simulink model "RobotX_September11"  (R2014a)
settings: Solver=FixedStepDiscrete  StartTime=0.0  StopTime=inf  FixedStep=.1  RelTol=1e-3
undefined symbols (not defined in the file): Com1, Com2, Com3, Com4, DiscIntNeverNeededParam
libraries: xpcseriallib x8, simulink x2, speedgoatlib_IO102 x1, slrtlib x1
(part 1 of 2)
settings Model: BufferReuse=off  Creator=wildcat  LastModifiedBy=wildcat
settings SolverCC: EnableConcurrentExecution=on
settings DataIOCC: SignalLoggingSaveFormat=ModelDataLogs
settings OptimizationCC: BlockReduction=off  OptimizeBlockIOStorage=off  BufferReuse=off  GlobalBufferReuse=off  ExpressionFolding=off  LocalBlockOutputs=off
settings DebuggingCC: UnderspecifiedInitializationDetection=Classic  StateNameClashWarn=warning
settings HardwareCC: ProdIntDivRoundTo=Zero  ProdEndianess=LittleEndian  ProdHWDeviceType=Generic->32-bit x86 compatible
settings RTWCC: SystemTargetFile=slrt.tlc  TemplateMakefile=slrt_default_tmf  Description=Simulink Real-Time  ProcessScript=slrt_make_rtw_hook  RTWCompilerOptimization=On
settings SimulinkRealTimeCC: GeneratePreprocessorConditionals=Disable all  EnableShiftOperators=on

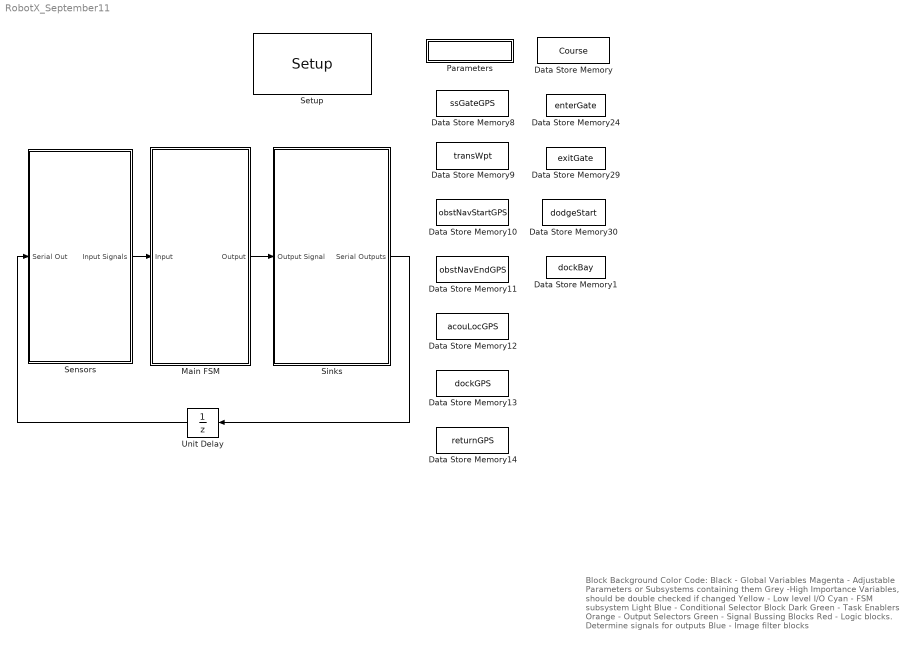
== system RobotX_September11 ==
  note: Block Background Color Code:
      | Black - Global Variables
      | Magenta - Adjustable Parameters or Subsystems containing them
      | Grey -High Importance Variables, should be double checked if changed
      | Yellow - Low level I/O
      | Cyan - FSM subsystem
      | Light Blue - Conditional Selector Block
      | Dark Green - Task Enablers
      | Orange - Output Selectors
      | Green - Signal Bussing Blocks
      | Red - Logic blocks. Determine signals for outputs
      | Blue - Image filter blocks
  Data Store Memory : DataStoreMemory  DataStoreName=Course  ReadBeforeWriteMsg=warning  WriteAfterWriteMsg=warning  WriteAfterReadMsg=warning
  Data Store Memory1 : DataStoreMemory  DataStoreName=dockBay  ReadBeforeWriteMsg=warning  WriteAfterWriteMsg=warning  WriteAfterReadMsg=warning
  Data Store Memory10 : DataStoreMemory  DataStoreName=obstNavStartGPS  ReadBeforeWriteMsg=warning  WriteAfterWriteMsg=warning  WriteAfterReadMsg=warning  InitialValue=zeros(1,2)
  Data Store Memory11 : DataStoreMemory  DataStoreName=obstNavEndGPS  ReadBeforeWriteMsg=warning  WriteAfterWriteMsg=warning  WriteAfterReadMsg=warning  InitialValue=zeros(1,2)
  Data Store Memory12 : DataStoreMemory  DataStoreName=acouLocGPS  ReadBeforeWriteMsg=warning  WriteAfterWriteMsg=warning  WriteAfterReadMsg=warning  InitialValue=zeros(1,2)
  Data Store Memory13 : DataStoreMemory  DataStoreName=dockGPS  ReadBeforeWriteMsg=warning  WriteAfterWriteMsg=warning  WriteAfterReadMsg=warning  InitialValue=zeros(1,2)
  Data Store Memory14 : DataStoreMemory  DataStoreName=returnGPS  ReadBeforeWriteMsg=warning  WriteAfterWriteMsg=warning  WriteAfterReadMsg=warning  InitialValue=zeros(1,2)
  Data Store Memory24 : DataStoreMemory  DataStoreName=enterGate  ReadBeforeWriteMsg=warning  WriteAfterWriteMsg=warning  WriteAfterReadMsg=warning
  Data Store Memory29 : DataStoreMemory  DataStoreName=exitGate  ReadBeforeWriteMsg=warning  WriteAfterWriteMsg=warning  WriteAfterReadMsg=warning
  Data Store Memory30 : DataStoreMemory  DataStoreName=dodgeStart  ReadBeforeWriteMsg=warning  WriteAfterWriteMsg=warning  WriteAfterReadMsg=warning
  Data Store Memory8 : DataStoreMemory  DataStoreName=ssGateGPS  ReadBeforeWriteMsg=warning  WriteAfterWriteMsg=warning  WriteAfterReadMsg=warning  InitialValue=zeros(1,2)
  Data Store Memory9 : DataStoreMemory  DataStoreName=transWpt  ReadBeforeWriteMsg=warning  WriteAfterWriteMsg=warning  WriteAfterReadMsg=warning  InitialValue=zeros(1,2)
  Main FSM : Subsystem
  Parameters : Subsystem
  Sensors : Subsystem
  Setup : speedgoatlib_IO102/Setup  group=Digital output setup  id=1  range=+-5V  cal=off  pciSlot=-1  adChannelMode=Multiple-channel (enter number of channels below)  adChannel=16  adCoupling=Differential  daChannel=[1,2,3,4]  daReset=[1]  daInitValue=[0]  diChannel=[1,2,3,4,5,6,7,8]  doChannel=[1,2,3,4,5,6,7,8]  doReset=[1]  doInitValue=[0]
  Sinks : Subsystem
  Unit Delay : UnitDelay  SampleTime=-1
  wires:
  Main FSM/1(Output) -> Sinks/1(Output Signal)
  Sensors/1(Input Signals) -> Main FSM/1(Input)
  Sinks/1(Serial Outputs) -> Unit Delay/1
  Unit Delay/1 -> Sensors/1(Serial Out)

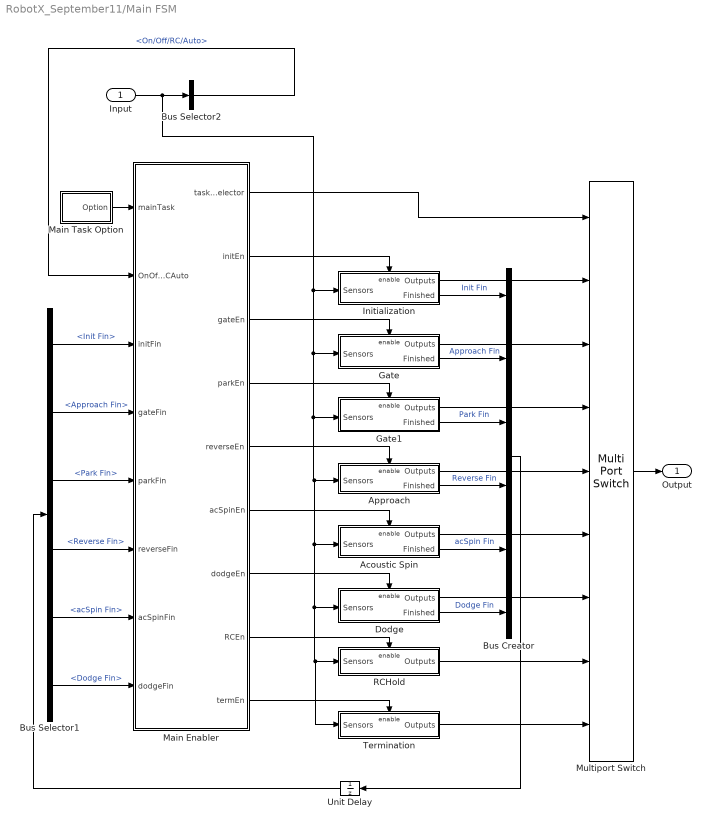
== system RobotX_September11/Main FSM ==
  Input : Inport
  Acoustic Spin : Subsystem  TreatAsAtomicUnit=on
  Approach : Subsystem  TreatAsAtomicUnit=on
  Bus Creator : BusCreator  Inputs=6
  Bus Selector1 : BusSelector  OutputSignals=Init Fin,Approach Fin,Park Fin,Reverse Fin,acSpin Fin,Dodge Fin
  Bus Selector2 : BusSelector  OutputSignals=LCM Message.On/Off/RC/Auto
  Dodge : Subsystem  TreatAsAtomicUnit=on
  Gate : Subsystem  TreatAsAtomicUnit=on
  Gate1 : Subsystem  TreatAsAtomicUnit=on
  Initialization : Subsystem
  Main Enabler : MATLAB Function  TreatAsAtomicUnit=on
  Main Task Option : Subsystem
  Multiport Switch : MultiPortSwitch  Inputs=8
  RCHold : Subsystem
  Termination : Subsystem  TreatAsAtomicUnit=on
  Unit Delay : UnitDelay  SampleTime=-1
  Output : Outport
  wires:
  Main Task Option/1(Option) -> Main Enabler/1(mainTask)
  Unit Delay/1 -> Bus Selector1/1
  Input/1 -> Gate/1(Sensors), Gate1/1(Sensors), Approach/1(Sensors), Acoustic Spin/1(Sensors), Dodge/1(Sensors), Termination/1(Sensors), RCHold/1(Sensors), Initialization/1(Sensors), Bus Selector2/1
  Bus Selector2/1 -> Main Enabler/2(OnOffRCAuto)  "<On/Off/RC/Auto>"
  Initialization/1(Outputs) -> Multiport Switch/2
  Gate/1(Outputs) -> Multiport Switch/3
  Approach/1(Outputs) -> Multiport Switch/5
  Dodge/1(Outputs) -> Multiport Switch/7
  RCHold/1(Outputs) -> Multiport Switch/8
  Termination/1(Outputs) -> Multiport Switch/9
  Bus Creator/1 -> Unit Delay/1
  Main Enabler/2(initEn) -> Initialization/Enable
  Main Enabler/3(gateEn) -> Gate/Enable
  Main Enabler/5(reverseEn) -> Approach/Enable
  Main Enabler/7(dodgeEn) -> Dodge/Enable
  Main Enabler/8(RCEn) -> RCHold/Enable
  Main Enabler/9(termEn) -> Termination/Enable
  Main Enabler/1(taskSelector) -> Multiport Switch/1
  Main Enabler/4(parkEn) -> Gate1/Enable
  Gate1/1(Outputs) -> Multiport Switch/4
  Initialization/2(Finished) -> Bus Creator/1  "Init Fin"
  Gate/2(Finished) -> Bus Creator/2  "Approach Fin"
  Gate1/2(Finished) -> Bus Creator/3  "Park Fin"
  Approach/2(Finished) -> Bus Creator/4  "Reverse Fin"
  Bus Selector1/1 -> Main Enabler/3(initFin)  "<Init Fin>"
  Bus Selector1/2 -> Main Enabler/4(gateFin)  "<Approach Fin>"
  Bus Selector1/3 -> Main Enabler/5(parkFin)  "<Park Fin>"
  Bus Selector1/4 -> Main Enabler/6(reverseFin)  "<Reverse Fin>"
  Bus Selector1/6 -> Main Enabler/8(dodgeFin)  "<Dodge Fin>"
  Multiport Switch/1 -> Output/1
  Acoustic Spin/2(Finished) -> Bus Creator/5  "acSpin Fin"
  Dodge/2(Finished) -> Bus Creator/6  "Dodge Fin"
  Acoustic Spin/1(Outputs) -> Multiport Switch/6
  Bus Selector1/5 -> Main Enabler/7(acSpinFin)  "<acSpin Fin>"
  Main Enabler/6(acSpinEn) -> Acoustic Spin/Enable

== system RobotX_September11/Parameters ==
  note: Course options are:
      | A, B and
      | otherwise (for testing,
      |  must be one character)
  CourseName : Constant  Value=uint8('B')  VectorParams1D=off
  GPS Points : Subsystem
  Write : DataStoreWrite  DataStoreName=Course
  wires:
  CourseName/1 -> Write/1

== system RobotX_September11/Sensors ==
  Serial Out : Inport
  Serial In : Subsystem
  Input Signals : Outport
  wires:
  Serial In/1(Serial In) -> Input Signals/1  "Sensors"
  Serial Out/1 -> Serial In/1(Serial Out)

== system RobotX_September11/Sinks ==
  Output Signal : Inport
  Bus Selector : BusSelector  OutputSignals=Outputs
  data log : Subsystem  Commented=on
  Serial Outputs : Outport
  wires:
  Output Signal/1 -> Bus Selector/1
  Bus Selector/1 -> Serial Outputs/1  "<Outputs>"

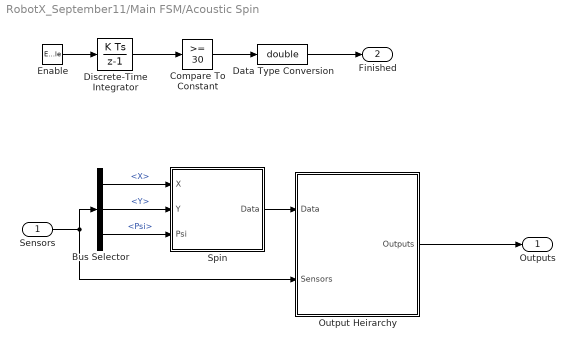
== system RobotX_September11/Main FSM/Acoustic Spin ==
  Sensors : Inport
  Enable : EnablePort  ShowOutputPort=on
  Bus Selector : BusSelector  OutputSignals=LCM Message.Pose.X,LCM Message.Pose.Y,LCM Message.Pose.Psi
  Compare To Constant : simulink/Logic and Bit Operations/Compare To Constant  relop=>=  const=30  OutDataTypeStr=boolean
  Data Type Conversion : DataTypeConversion  OutDataTypeStr=double
  Discrete-Time Integrator : DiscreteIntegrator  SampleTime=0.1  ICPrevOutput=DiscIntNeverNeededParam  ICPrevScaledInput=DiscIntNeverNeededParam
  Output Heirarchy : Subsystem
  Spin : MATLAB Function  TreatAsAtomicUnit=on
  Outputs : Outport
  Finished : Outport  Port=2
  wires:
  Sensors/1 -> Output Heirarchy/2(Sensors), Bus Selector/1
  Bus Selector/1 -> Spin/1(X)  "<X>"
  Bus Selector/3 -> Spin/3(Psi)  "<Psi>"
  Bus Selector/2 -> Spin/2(Y)  "<Y>"
  Spin/1(Data) -> Output Heirarchy/1(Data)
  Output Heirarchy/1(Outputs) -> Outputs/1
  Compare To Constant/1 -> Data Type Conversion/1
  Enable/1 -> Discrete-Time Integrator/1
  Data Type Conversion/1 -> Finished/1
  Discrete-Time Integrator/1 -> Compare To Constant/1

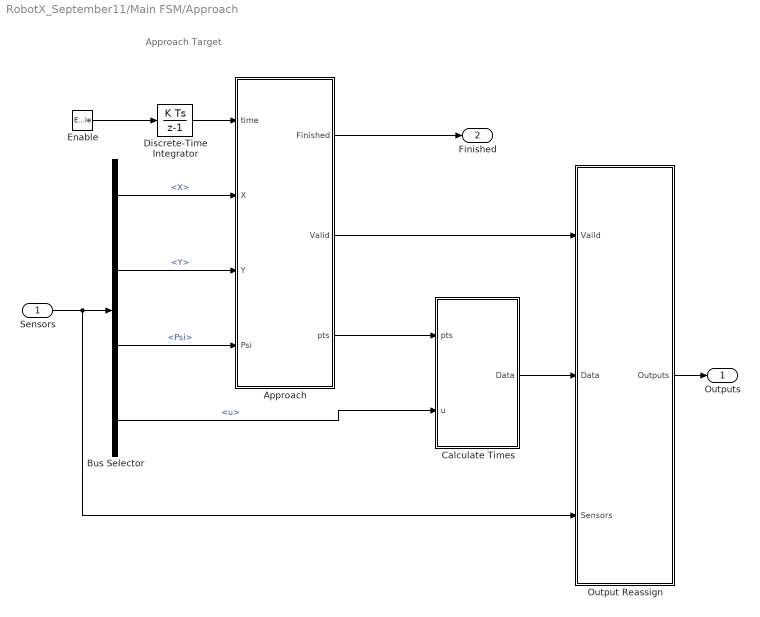
== system RobotX_September11/Main FSM/Approach ==
  note: Approach Target
  Sensors : Inport
  Enable : EnablePort  ShowOutputPort=on
  Approach : MATLAB Function  TreatAsAtomicUnit=on
  Bus Selector : BusSelector  OutputSignals=LCM Message.Pose.X,LCM Message.Pose.Y,LCM Message.Pose.Psi,LCM Message.Velocity.u
  Calculate Times : MATLAB Function  TreatAsAtomicUnit=on
  Discrete-Time Integrator : DiscreteIntegrator  SampleTime=0.1  ICPrevOutput=DiscIntNeverNeededParam  ICPrevScaledInput=DiscIntNeverNeededParam
  Output Reassign : Subsystem
  Outputs : Outport
  Finished : Outport  Port=2
  wires:
  Output Reassign/1(Outputs) -> Outputs/1
  Approach/1(Finished) -> Finished/1
  Sensors/1 -> Output Reassign/3(Sensors), Bus Selector/1
  Enable/1 -> Discrete-Time Integrator/1
  Discrete-Time Integrator/1 -> Approach/1(time)
  Bus Selector/3 -> Approach/4(Psi)  "<Psi>"
  Bus Selector/2 -> Approach/3(Y)  "<Y>"
  Bus Selector/1 -> Approach/2(X)  "<X>"
  Bus Selector/4 -> Calculate Times/2(u)  "<u>"
  Approach/3(pts) -> Calculate Times/1(pts)
  Calculate Times/1(Data) -> Output Reassign/2(Data)
  Approach/2(Valid) -> Output Reassign/1(Vaild)

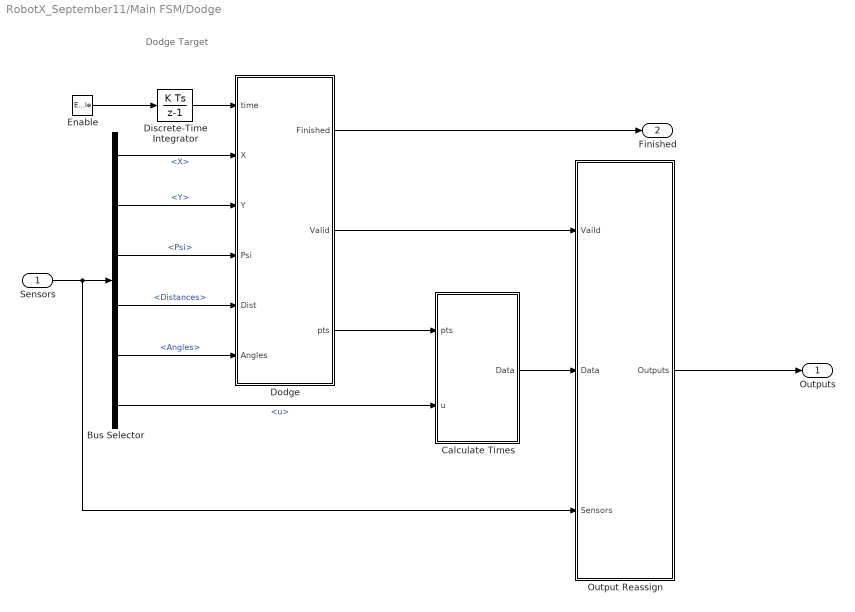
== system RobotX_September11/Main FSM/Dodge ==
  note: Dodge Target
  Sensors : Inport
  Enable : EnablePort  ShowOutputPort=on
  Bus Selector : BusSelector  OutputSignals=LCM Message.Pose.X,LCM Message.Pose.Y,LCM Message.Pose.Psi,Lidar Data Input.Landmarks.Distances,Lidar Data Input.Landmarks.Angles,LCM Message.Velocity.u
  Calculate Times : MATLAB Function  TreatAsAtomicUnit=on
  Discrete-Time Integrator : DiscreteIntegrator  SampleTime=0.1  ICPrevOutput=DiscIntNeverNeededParam  ICPrevScaledInput=DiscIntNeverNeededParam
  Dodge : MATLAB Function  TreatAsAtomicUnit=on
  Output Reassign : Subsystem
  Outputs : Outport
  Finished : Outport  Port=2
  wires:
  Output Reassign/1(Outputs) -> Outputs/1
  Dodge/1(Finished) -> Finished/1
  Sensors/1 -> Output Reassign/3(Sensors), Bus Selector/1
  Enable/1 -> Discrete-Time Integrator/1
  Discrete-Time Integrator/1 -> Dodge/1(time)
  Bus Selector/3 -> Dodge/4(Psi)  "<Psi>"
  Bus Selector/2 -> Dodge/3(Y)  "<Y>"
  Bus Selector/4 -> Dodge/5(Dist)  "<Distances>"
  Bus Selector/5 -> Dodge/6(Angles)  "<Angles>"
  Bus Selector/1 -> Dodge/2(X)  "<X>"
  Bus Selector/6 -> Calculate Times/2(u)  "<u>"
  Dodge/3(pts) -> Calculate Times/1(pts)
  Calculate Times/1(Data) -> Output Reassign/2(Data)
  Dodge/2(Valid) -> Output Reassign/1(Vaild)

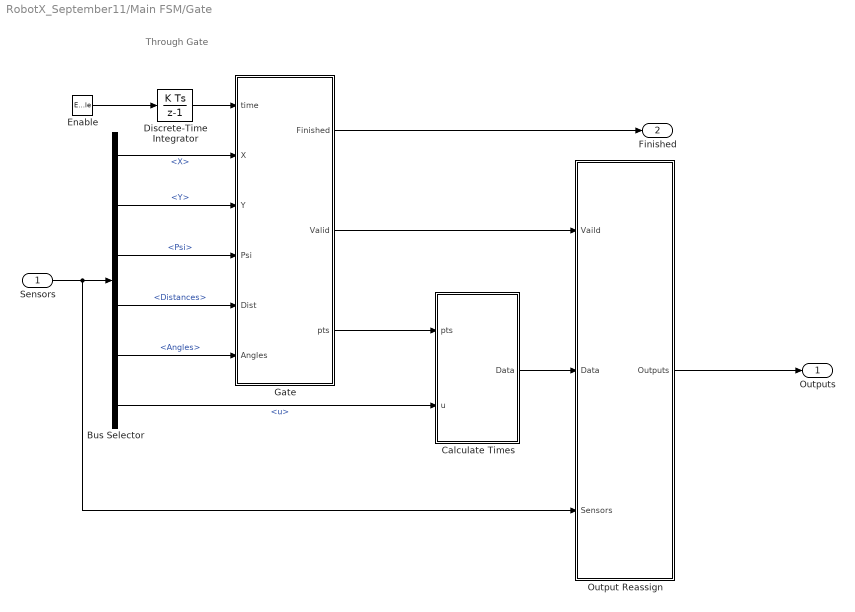
== system RobotX_September11/Main FSM/Gate ==
  note: Through Gate
  Sensors : Inport
  Enable : EnablePort  ShowOutputPort=on
  Bus Selector : BusSelector  OutputSignals=LCM Message.Pose.X,LCM Message.Pose.Y,LCM Message.Pose.Psi,Lidar Data Input.Landmarks.Distances,Lidar Data Input.Landmarks.Angles,LCM Message.Velocity.u
  Calculate Times : MATLAB Function  TreatAsAtomicUnit=on
  Discrete-Time Integrator : DiscreteIntegrator  SampleTime=0.1  ICPrevOutput=DiscIntNeverNeededParam  ICPrevScaledInput=DiscIntNeverNeededParam
  Gate : MATLAB Function  TreatAsAtomicUnit=on
  Output Reassign : Subsystem
  Outputs : Outport
  Finished : Outport  Port=2
  wires:
  Output Reassign/1(Outputs) -> Outputs/1
  Gate/1(Finished) -> Finished/1
  Sensors/1 -> Output Reassign/3(Sensors), Bus Selector/1
  Enable/1 -> Discrete-Time Integrator/1
  Discrete-Time Integrator/1 -> Gate/1(time)
  Bus Selector/3 -> Gate/4(Psi)  "<Psi>"
  Bus Selector/2 -> Gate/3(Y)  "<Y>"
  Bus Selector/4 -> Gate/5(Dist)  "<Distances>"
  Bus Selector/5 -> Gate/6(Angles)  "<Angles>"
  Bus Selector/1 -> Gate/2(X)  "<X>"
  Bus Selector/6 -> Calculate Times/2(u)  "<u>"
  Gate/3(pts) -> Calculate Times/1(pts)
  Calculate Times/1(Data) -> Output Reassign/2(Data)
  Gate/2(Valid) -> Output Reassign/1(Vaild)

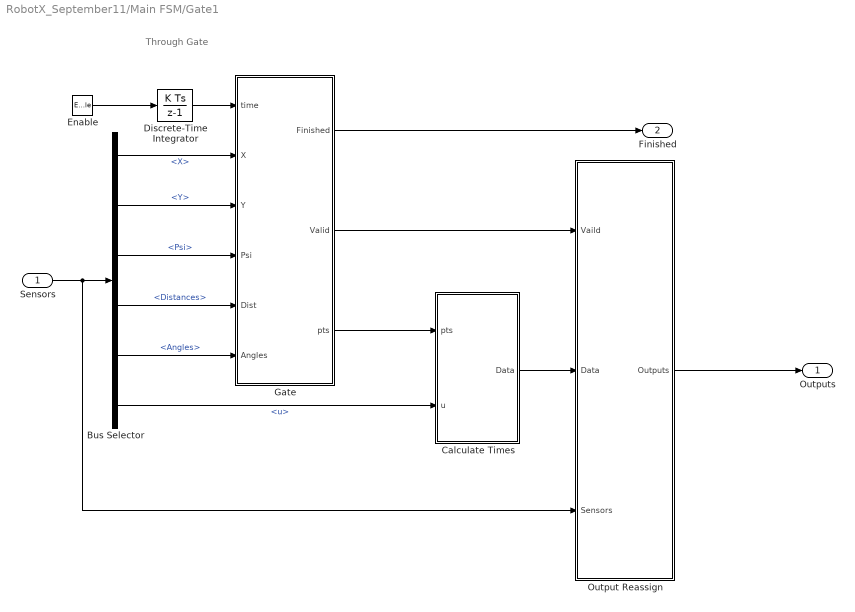
== system RobotX_September11/Main FSM/Gate1 ==
  note: Through Gate
  Sensors : Inport
  Enable : EnablePort  ShowOutputPort=on
  Bus Selector : BusSelector  OutputSignals=LCM Message.Pose.X,LCM Message.Pose.Y,LCM Message.Pose.Psi,Lidar Data Input.Landmarks.Distances,Lidar Data Input.Landmarks.Angles,LCM Message.Velocity.u
  Calculate Times : MATLAB Function  TreatAsAtomicUnit=on
  Discrete-Time Integrator : DiscreteIntegrator  SampleTime=0.1  ICPrevOutput=DiscIntNeverNeededParam  ICPrevScaledInput=DiscIntNeverNeededParam
  Gate : MATLAB Function  TreatAsAtomicUnit=on
  Output Reassign : Subsystem
  Outputs : Outport
  Finished : Outport  Port=2
  wires:
  Output Reassign/1(Outputs) -> Outputs/1
  Gate/1(Finished) -> Finished/1
  Sensors/1 -> Output Reassign/3(Sensors), Bus Selector/1
  Enable/1 -> Discrete-Time Integrator/1
  Discrete-Time Integrator/1 -> Gate/1(time)
  Bus Selector/3 -> Gate/4(Psi)  "<Psi>"
  Bus Selector/2 -> Gate/3(Y)  "<Y>"
  Bus Selector/4 -> Gate/5(Dist)  "<Distances>"
  Bus Selector/5 -> Gate/6(Angles)  "<Angles>"
  Bus Selector/1 -> Gate/2(X)  "<X>"
  Bus Selector/6 -> Calculate Times/2(u)  "<u>"
  Gate/3(pts) -> Calculate Times/1(pts)
  Calculate Times/1(Data) -> Output Reassign/2(Data)
  Gate/2(Valid) -> Output Reassign/1(Vaild)

== system RobotX_September11/Main FSM/Initialization ==
  Sensors : Inport
  Enable : EnablePort  ShowOutputPort=on
  Compare To Constant : simulink/Logic and Bit Operations/Compare To Constant  relop=>=  const=50  OutDataTypeStr=boolean
  Data Type Conversion : DataTypeConversion  OutDataTypeStr=double
  Discrete-Time Integrator : DiscreteIntegrator  SampleTime=0.1  ICPrevOutput=DiscIntNeverNeededParam  ICPrevScaledInput=DiscIntNeverNeededParam
  Output Heirarchy : Subsystem
  Outputs : Outport
  Finished : Outport  Port=2
  wires:
  Sensors/1 -> Output Heirarchy/1(Sensors)
  Output Heirarchy/1(Outputs) -> Outputs/1
  Compare To Constant/1 -> Data Type Conversion/1
  Enable/1 -> Discrete-Time Integrator/1
  Discrete-Time Integrator/1 -> Compare To Constant/1
  Data Type Conversion/1 -> Finished/1

== system RobotX_September11/Main FSM/Main Task Option ==
  note: Main Task Options
  Message Composer : MATLAB Function  TreatAsAtomicUnit=on
  Test Comms Option : Constant  Value=uint8(' ')  SampleTime=0.1
  Option : Outport
  wires:
  Test Comms Option/1 -> Message Composer/1(taskStrInit)
  Message Composer/1(taskStrAdj) -> Option/1

== system RobotX_September11/Main FSM/RCHold ==
  Sensors : Inport
  Enable : EnablePort
  Bus Selector : BusSelector  Commented=on  OutputSignals=LCM Message.Pose.X,LCM Message.Pose.Y,LCM Message.Pose.Psi
  Direct Control : Subsystem
  Output Heirarchy : Subsystem  Commented=on
  Set Pose : MATLAB Function  Commented=on  TreatAsAtomicUnit=on
  Outputs : Outport
  wires:
  Direct Control/1(Outputs) -> Outputs/1
  Bus Selector/1 -> Set Pose/1(X)  "<X>"
  Bus Selector/3 -> Set Pose/3(Psi)  "<Psi>"
  Bus Selector/2 -> Set Pose/2(Y)  "<Y>"
  Set Pose/1(Data) -> Output Heirarchy/1(Data)
  Sensors/1 -> Direct Control/1(Sensors), Bus Selector/1

== system RobotX_September11/Main FSM/Termination ==
  Sensors : Inport
  Enable : EnablePort
  Bus Selector : BusSelector  OutputSignals=LCM Message.Pose.X,LCM Message.Pose.Y,LCM Message.Pose.Psi,Lidar Data Input.Landmarks.Distances,Lidar Data Input.Landmarks.Angles
  Direct Control : Subsystem  Commented=on
  Output Heirarchy : Subsystem
  Point : MATLAB Function  TreatAsAtomicUnit=on
  Outputs : Outport
  wires:
  Sensors/1 -> Output Heirarchy/2(Sensors), Bus Selector/1
  Bus Selector/1 -> Point/1(X)  "<X>"
  Bus Selector/3 -> Point/3(Psi)  "<Psi>"
  Bus Selector/2 -> Point/2(Y)  "<Y>"
  Point/1(Data) -> Output Heirarchy/1(Data)
  Output Heirarchy/1(Outputs) -> Outputs/1
  Bus Selector/4 -> Point/4(Dist)  "<Distances>"
  Bus Selector/5 -> Point/5(Angle)  "<Angles>"

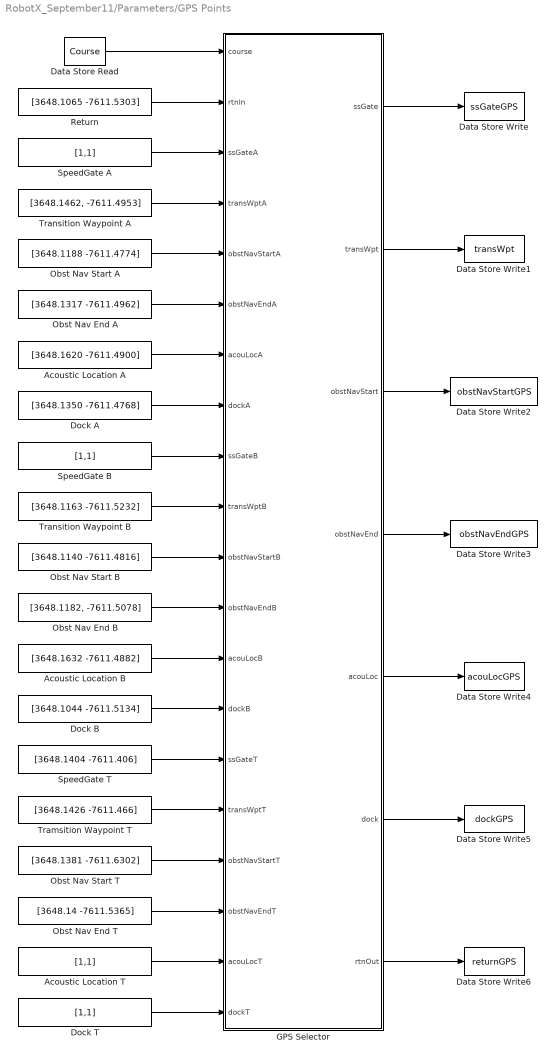
== system RobotX_September11/Parameters/GPS Points ==
  Acoustic Location A : Constant  Value=[3648.1620 -7611.4900]  SampleTime=0.1
  Acoustic Location B : Constant  Value=[3648.1632 -7611.4882]  SampleTime=0.1
  Acoustic Location T : Constant  Value=[1,1]  SampleTime=0.1
  Data Store Read : DataStoreRead  DialogController=Simulink.DDGSource  DataStoreName=Course  SampleTime=0.1
  Data Store Write : DataStoreWrite  DialogController=Simulink.DDGSource  DataStoreName=ssGateGPS
  Data Store Write1 : DataStoreWrite  DataStoreName=transWpt
  Data Store Write2 : DataStoreWrite  DataStoreName=obstNavStartGPS
  Data Store Write3 : DataStoreWrite  DataStoreName=obstNavEndGPS
  Data Store Write4 : DataStoreWrite  DataStoreName=acouLocGPS
  Data Store Write5 : DataStoreWrite  DataStoreName=dockGPS
  Data Store Write6 : DataStoreWrite  DataStoreName=returnGPS
  Dock A : Constant  Value=[3648.1350 -7611.4768]  SampleTime=0.1
  Dock B : Constant  Value=[3648.1044 -7611.5134]  SampleTime=0.1
  Dock T : Constant  Value=[1,1]  SampleTime=0.1
  GPS Selector : MATLAB Function  TreatAsAtomicUnit=on
  Obst Nav End A : Constant  Value=[3648.1317 -7611.4962]  SampleTime=0.1
  Obst Nav End B : Constant  Value=[3648.1182, -7611.5078]  SampleTime=0.1
  Obst Nav End T : Constant  Value=[3648.14 -7611.5365]  SampleTime=0.1
  Obst Nav Start A : Constant  Value=[3648.1188 -7611.4774]  SampleTime=0.1
  Obst Nav Start B : Constant  Value=[3648.1140 -7611.4816]  SampleTime=0.1
  Obst Nav Start T : Constant  Value=[3648.1381 -7611.6302]  SampleTime=0.1
  Return : Constant  Value=[3648.1065 -7611.5303]  SampleTime=0.1
  SpeedGate A : Constant  Value=[1,1]  SampleTime=0.1
  SpeedGate B : Constant  Value=[1,1]  SampleTime=0.1
  SpeedGate T : Constant  Value=[3648.1404 -7611.406]  SampleTime=0.1
  Tramsition Waypoint T : Constant  Value=[3648.1426 -7611.466]  SampleTime=0.1
  Transition Waypoint A : Constant  Value=[3648.1462, -7611.4953]  SampleTime=0.1
  Transition Waypoint B : Constant  Value=[3648.1163 -7611.5232]  SampleTime=0.1
  wires:
  Data Store Read/1 -> GPS Selector/1(course)
  Return/1 -> GPS Selector/2(rtnIn)
  SpeedGate A/1 -> GPS Selector/3(ssGateA)
  Transition Waypoint A/1 -> GPS Selector/4(transWptA)
  Obst Nav Start A/1 -> GPS Selector/5(obstNavStartA)
  Obst Nav End A/1 -> GPS Selector/6(obstNavEndA)
  SpeedGate T/1 -> GPS Selector/15(ssGateT)
  Acoustic Location T/1 -> GPS Selector/19(acouLocT)
  Tramsition Waypoint T/1 -> GPS Selector/16(transWptT)
  Dock A/1 -> GPS Selector/8(dockA)
  Dock T/1 -> GPS Selector/20(dockT)
  Obst Nav End T/1 -> GPS Selector/18(obstNavEndT)
  Obst Nav Start T/1 -> GPS Selector/17(obstNavStartT)
  Obst Nav Start B/1 -> GPS Selector/11(obstNavStartB)
  Obst Nav End B/1 -> GPS Selector/12(obstNavEndB)
  Acoustic Location A/1 -> GPS Selector/7(acouLocA)
  Acoustic Location B/1 -> GPS Selector/13(acouLocB)
  Dock B/1 -> GPS Selector/14(dockB)
  SpeedGate B/1 -> GPS Selector/9(ssGateB)
  Transition Waypoint B/1 -> GPS Selector/10(transWptB)
  GPS Selector/1(ssGate) -> Data Store Write/1
  GPS Selector/2(transWpt) -> Data Store Write1/1
  GPS Selector/3(obstNavStart) -> Data Store Write2/1
  GPS Selector/4(obstNavEnd) -> Data Store Write3/1
  GPS Selector/5(acouLoc) -> Data Store Write4/1
  GPS Selector/6(dock) -> Data Store Write5/1
  GPS Selector/7(rtnOut) -> Data Store Write6/1

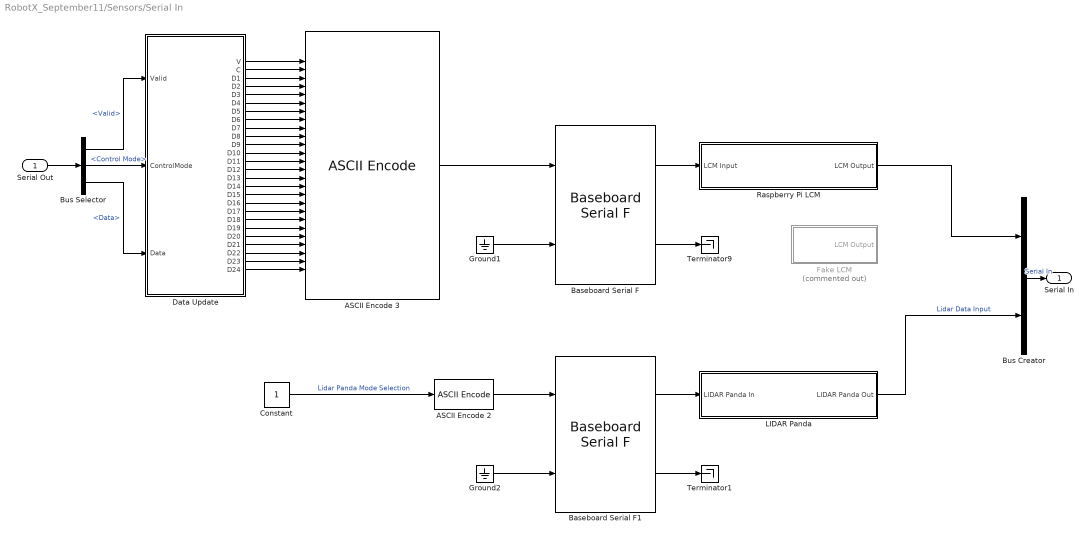
== system RobotX_September11/Sensors/Serial In ==
  Serial Out : Inport
  " Raspberry Pi LCM" : Subsystem
  ASCII Encode 2 : xpcseriallib/ASCII Encode   format=SGTask:%d \r\n  nvars=1  maxlength=128  vartypes={ 'double' }
  ASCII Encode 3 : xpcseriallib/ASCII Encode   format="{\"Valid\":%d, \"Mode\":%d, \"A\":%5.2f, \"B\":%5.2f, \"C\":%4.2f, \"D\":%5.2f, \"E\":%5.2f, \"F\":%4.2f, \"G\":%5.2f, \"H\":%5.2f, \"I\":%4.2f, \"J\":%5.2f, \"K\":%5.2f, \"L\":%4.2f, \"M\":%5.2f, \"N\":%5.2f, \"O\":%4.2f, \"P\":%5.2f, \"Q\":%5.2f, \"R\":%4.2f, \"S\":%5.2f, \"T\":%5.2f, \"U\":%4.2f, \"V\":%5.2f, \"W\":%5.2f, \"X\":%4.2f} \\r\\n"  nvars=26  maxlength=300  vartypes={ 'double' }
  Baseboard Serial F : xpcseriallib/Mainboard/Baseboard Serial F  group=Basic Setup  port=1  irqnum=4  saddr1=0x3f8  saddr2=0x3e8  config=Com1/Com3  baud1=115200  parity1=Even  ndata1=7  nstop1=1  fifomode1=64 deep  rlevel1=quarter full  automode1=on  xmtfifosize1=1024  xmtdatatype1=8 bit uint null terminated  rcvfifosize1=1024  baud2=115200  parity2=Even  ndata2=7  nstop2=1  fifomode2=64 deep  rlevel2=1  automode2=on  xmtfifosize2=1024  xmtdatatype2=8 bit uint null terminated  rcvfifosize2=1024
  Baseboard Serial F1 : xpcseriallib/Mainboard/Baseboard Serial F  group=Basic Setup  port=2  irqnum=4  saddr1=0x3f8  saddr2=0x3e8  config=Com2/Com4  baud1=115200  parity1=Even  ndata1=7  nstop1=1  fifomode1=64 deep  rlevel1=quarter full  automode1=on  xmtfifosize1=1024  xmtdatatype1=8 bit uint null terminated  rcvfifosize1=1024  baud2=115200  parity2=Even  ndata2=7  nstop2=1  fifomode2=64 deep  rlevel2=quarter full  automode2=on  xmtfifosize2=1024  xmtdatatype2=8 bit uint null terminated  rcvfifosize2=1024
  Bus Creator : BusCreator  Inputs=2
  Bus Selector : BusSelector  OutputSignals=Valid,Control Mode,Data
  Constant : Constant
  Data Update : MATLAB Function  TreatAsAtomicUnit=on
  Fake LCM : Subsystem  Commented=on
  Ground1 : Ground
  Ground2 : Ground
  LIDAR Panda : Subsystem
  Terminator1 : Terminator
  Terminator9 : Terminator
  Serial In : Outport
  wires:
  Bus Creator/1 -> Serial In/1  "Serial In"
  Baseboard Serial F1/1 -> LIDAR Panda/1(LIDAR Panda In)
  LIDAR Panda/1(LIDAR Panda Out) -> Bus Creator/2  "Lidar Data Input"
  ASCII Encode 2/1 -> Baseboard Serial F1/1
  Constant/1 -> ASCII Encode 2/1  "Lidar Panda Mode Selection"
  Baseboard Serial F/2 -> Terminator9/1
  Serial Out/1 -> Bus Selector/1
  Ground1/1 -> Baseboard Serial F/2
  Baseboard Serial F/1 -> " Raspberry Pi LCM"/1(LCM Input)
  Baseboard Serial F1/2 -> Terminator1/1
  ASCII Encode 3/1 -> Baseboard Serial F/1
  " Raspberry Pi LCM"/1(LCM Output) -> Bus Creator/1
  Ground2/1 -> Baseboard Serial F1/2
  Data Update/9(D7) -> ASCII Encode 3/9
  Data Update/11(D9) -> ASCII Encode 3/11
  Data Update/3(D1) -> ASCII Encode 3/3
  Data Update/6(D4) -> ASCII Encode 3/6
  Data Update/7(D5) -> ASCII Encode 3/7
  Data Update/2(C) -> ASCII Encode 3/2
  Data Update/5(D3) -> ASCII Encode 3/5
  Data Update/4(D2) -> ASCII Encode 3/4
  Data Update/13(D11) -> ASCII Encode 3/13
  Data Update/14(D12) -> ASCII Encode 3/14
  Data Update/1(V) -> ASCII Encode 3/1
  Data Update/12(D10) -> ASCII Encode 3/12
  Data Update/10(D8) -> ASCII Encode 3/10
  Data Update/8(D6) -> ASCII Encode 3/8
  Bus Selector/1 -> Data Update/1(Valid)  "<Valid>"
  Bus Selector/2 -> Data Update/2(ControlMode)  "<Control Mode>"
  Bus Selector/3 -> Data Update/3(Data)  "<Data>"
  Data Update/24(D22) -> ASCII Encode 3/24
  Data Update/26(D24) -> ASCII Encode 3/26
  Data Update/18(D16) -> ASCII Encode 3/18
  Data Update/23(D21) -> ASCII Encode 3/23
  Data Update/22(D20) -> ASCII Encode 3/22
  Data Update/21(D19) -> ASCII Encode 3/21
  Data Update/19(D17) -> ASCII Encode 3/19
  Data Update/17(D15) -> ASCII Encode 3/17
  Data Update/16(D14) -> ASCII Encode 3/16
  Data Update/25(D23) -> ASCII Encode 3/25
  Data Update/20(D18) -> ASCII Encode 3/20
  Data Update/15(D13) -> ASCII Encode 3/15

== system RobotX_September11/Sinks/data log ==
  note: need to play with the boat to figure out how this works properly
  Output signal : Inport
  "Scope " : slrtlib/Displays and Logging/Scope   scopeno=1  scopetype=File  autostart=on  viewmode=Graphical redraw  formatstr='%15.6f'  grid=on  ylimits=[0,0]  nosamples=250  noprepostsamples=0  interleave=1  triggermode=Signal triggering  triggersignal=1  trigsignalfromport=on  triggerlevel=1  triggerslope=Rising  triggerscope=1  triggersample=0  filename=data.dat  mode=Lazy  writesize=512  autorestart=off  dynamicfilemode=off  maxwritefilesize=512*1024^2
  wires:
  Output signal/1 -> ?

== system RobotX_September11/Main FSM/Acoustic Spin/Output Heirarchy ==
  Data : Inport
  Sensors : Inport  Port=2
  Bus Creator1 : BusCreator  Inputs=3
  Bus Creator4 : BusCreator  Inputs=2
  Constant1 : Constant
  Constant2 : Constant
  Data Type Conversion : DataTypeConversion  OutDataTypeStr=double
  Outputs : Outport
  wires:
  Bus Creator1/1 -> Bus Creator4/1  "Outputs"
  Sensors/1 -> Bus Creator4/2  "Sensors"
  Bus Creator4/1 -> Outputs/1  "Output Signals"
  Constant1/1 -> Bus Creator1/2  "Control Mode"
  Data/1 -> Bus Creator1/3  "Data"
  Data Type Conversion/1 -> Bus Creator1/1  "Valid"
  Constant2/1 -> Data Type Conversion/1  "Valid"

== system RobotX_September11/Main FSM/Approach/Output Reassign ==
  Vaild : Inport
  Data : Inport  Port=2
  Sensors : Inport  Port=3
  Bus Creator1 : BusCreator  Inputs=3
  Bus Creator4 : BusCreator  Inputs=2
  Constant1 : Constant  Value=0
  Outputs : Outport
  wires:
  Bus Creator1/1 -> Bus Creator4/1  "Outputs"
  Sensors/1 -> Bus Creator4/2  "Sensors"
  Bus Creator4/1 -> Outputs/1  "Output Signals"
  Vaild/1 -> Bus Creator1/1  "Valid"
  Constant1/1 -> Bus Creator1/2  "Control Mode"
  Data/1 -> Bus Creator1/3  "Data"

== system RobotX_September11/Main FSM/Dodge/Output Reassign ==
  Vaild : Inport
  Data : Inport  Port=2
  Sensors : Inport  Port=3
  Bus Creator1 : BusCreator  Inputs=3
  Bus Creator4 : BusCreator  Inputs=2
  Constant1 : Constant  Value=0
  Outputs : Outport
  wires:
  Bus Creator1/1 -> Bus Creator4/1  "Outputs"
  Sensors/1 -> Bus Creator4/2  "Sensors"
  Bus Creator4/1 -> Outputs/1  "Output Signals"
  Vaild/1 -> Bus Creator1/1  "Valid"
  Constant1/1 -> Bus Creator1/2  "Control Mode"
  Data/1 -> Bus Creator1/3  "Data"

== system RobotX_September11/Main FSM/Gate/Output Reassign ==
  Vaild : Inport
  Data : Inport  Port=2
  Sensors : Inport  Port=3
  Bus Creator1 : BusCreator  Inputs=3
  Bus Creator4 : BusCreator  Inputs=2
  Constant1 : Constant  Value=0
  Outputs : Outport
  wires:
  Bus Creator1/1 -> Bus Creator4/1  "Outputs"
  Sensors/1 -> Bus Creator4/2  "Sensors"
  Bus Creator4/1 -> Outputs/1  "Output Signals"
  Vaild/1 -> Bus Creator1/1  "Valid"
  Constant1/1 -> Bus Creator1/2  "Control Mode"
  Data/1 -> Bus Creator1/3  "Data"

== system RobotX_September11/Main FSM/Gate1/Output Reassign ==
  Vaild : Inport
  Data : Inport  Port=2
  Sensors : Inport  Port=3
  Bus Creator1 : BusCreator  Inputs=3
  Bus Creator4 : BusCreator  Inputs=2
  Constant1 : Constant  Value=0
  Outputs : Outport
  wires:
  Bus Creator1/1 -> Bus Creator4/1  "Outputs"
  Sensors/1 -> Bus Creator4/2  "Sensors"
  Bus Creator4/1 -> Outputs/1  "Output Signals"
  Vaild/1 -> Bus Creator1/1  "Valid"
  Constant1/1 -> Bus Creator1/2  "Control Mode"
  Data/1 -> Bus Creator1/3  "Data"

== system RobotX_September11/Main FSM/Initialization/Output Heirarchy ==
  Sensors : Inport
  Bus Creator1 : BusCreator  Inputs=3
  Bus Creator4 : BusCreator  Inputs=2
  Constant : Constant  Value=0
  Constant1 : Constant  Value=0
  Constant2 : Constant  Value=zeros(12,1)
  Outputs : Outport
  wires:
  Bus Creator1/1 -> Bus Creator4/1  "Outputs"
  Sensors/1 -> Bus Creator4/2  "Sensors"
  Bus Creator4/1 -> Outputs/1  "Output Signals"
  Constant/1 -> Bus Creator1/1  "Valid"
  Constant1/1 -> Bus Creator1/2  "Control Mode"
  Constant2/1 -> Bus Creator1/3  "Data"

== system RobotX_September11/Main FSM/RCHold/Direct Control ==
  Sensors : Inport
  Bus Creator1 : BusCreator  Inputs=3
  Bus Creator4 : BusCreator  Inputs=2
  Constant : Constant
  Constant1 : Constant  Value=2
  Constant2 : Constant  Value=[0; 0; 0; 0; 0; 0; 0; 0; 0; 0; 0; 0]
  Outputs : Outport
  wires:
  Bus Creator1/1 -> Bus Creator4/1  "Outputs"
  Sensors/1 -> Bus Creator4/2  "Sensors"
  Bus Creator4/1 -> Outputs/1  "Output Signals"
  Constant/1 -> Bus Creator1/1  "Valid"
  Constant1/1 -> Bus Creator1/2  "Control Mode"
  Constant2/1 -> Bus Creator1/3  "Data"

== system RobotX_September11/Main FSM/RCHold/Output Heirarchy ==
  Data : Inport
  Sensors : Inport  Port=2
  Bus Creator1 : BusCreator  Inputs=3
  Bus Creator4 : BusCreator  Inputs=2
  Constant1 : Constant
  Constant2 : Constant
  Data Type Conversion : DataTypeConversion  OutDataTypeStr=double
  Outputs : Outport
  wires:
  Bus Creator1/1 -> Bus Creator4/1  "Outputs"
  Sensors/1 -> Bus Creator4/2  "Sensors"
  Bus Creator4/1 -> Outputs/1  "Output Signals"
  Constant1/1 -> Bus Creator1/2  "Control Mode"
  Data/1 -> Bus Creator1/3  "Data"
  Data Type Conversion/1 -> Bus Creator1/1  "Valid"
  Constant2/1 -> Data Type Conversion/1  "Valid"

== system RobotX_September11/Main FSM/Termination/Direct Control ==
  Sensors : Inport
  Bus Creator1 : BusCreator  Inputs=3
  Bus Creator4 : BusCreator  Inputs=2
  Constant : Constant
  Constant1 : Constant  Value=2
  Constant2 : Constant  Value=[0; 0; 0; 0; 0; 0; 0; 0; 0; 0; 0; 0]
  Outputs : Outport
  wires:
  Bus Creator1/1 -> Bus Creator4/1  "Outputs"
  Sensors/1 -> Bus Creator4/2  "Sensors"
  Bus Creator4/1 -> Outputs/1  "Output Signals"
  Constant/1 -> Bus Creator1/1  "Valid"
  Constant1/1 -> Bus Creator1/2  "Control Mode"
  Constant2/1 -> Bus Creator1/3  "Data"

== system RobotX_September11/Main FSM/Termination/Output Heirarchy ==
  Data : Inport
  Sensors : Inport  Port=2
  Bus Creator1 : BusCreator  Inputs=3
  Bus Creator4 : BusCreator  Inputs=2
  Constant1 : Constant
  Constant2 : Constant
  Data Type Conversion : DataTypeConversion  OutDataTypeStr=double
  Outputs : Outport
  wires:
  Bus Creator1/1 -> Bus Creator4/1  "Outputs"
  Sensors/1 -> Bus Creator4/2  "Sensors"
  Bus Creator4/1 -> Outputs/1  "Output Signals"
  Constant1/1 -> Bus Creator1/2  "Control Mode"
  Data/1 -> Bus Creator1/3  "Data"
  Data Type Conversion/1 -> Bus Creator1/1  "Valid"
  Constant2/1 -> Data Type Conversion/1  "Valid"

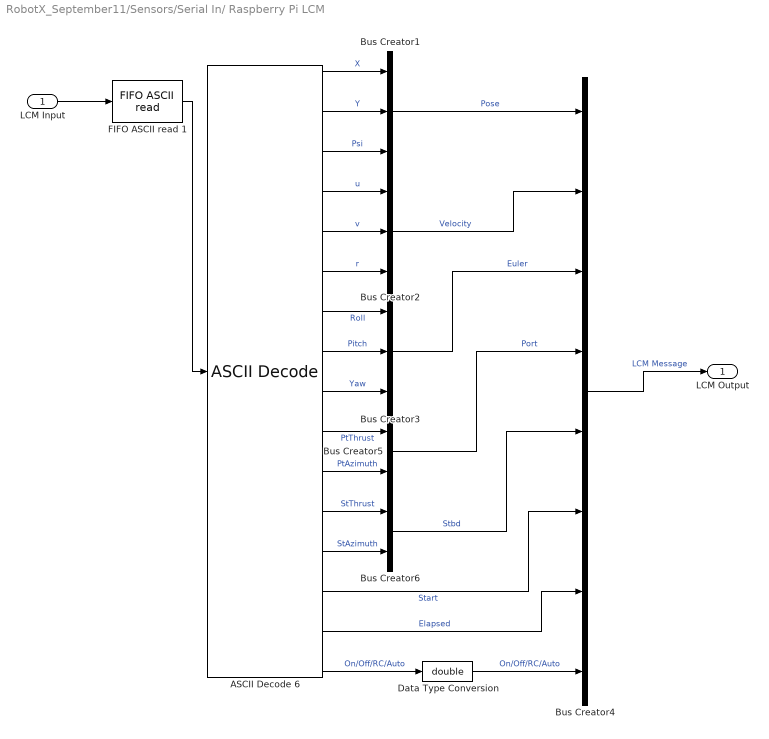
== system RobotX_September11/Sensors/Serial In/ Raspberry Pi LCM ==
  LCM Input : Inport
  ASCII Decode 6 : xpcseriallib/ASCII Decode   format=P1:%f P2:%f P3:%f V1:%f V2:%f V3:%f E1:%f E2:%f E3:%f Pt1:%f Pt2:%f St1:%f St2:%f Start:%f Elapsed:%f RC:%d \r\n  nvars=16  vartypes={}
  Bus Creator1 : BusCreator  Inputs=3
  Bus Creator2 : BusCreator  Inputs=3
  Bus Creator3 : BusCreator  Inputs=3
  Bus Creator4 : BusCreator  Inputs=8
  Bus Creator5 : BusCreator  Inputs=2
  Bus Creator6 : BusCreator  Inputs=2
  Data Type Conversion : DataTypeConversion  OutDataTypeStr=double
  FIFO ASCII read 1 : xpcseriallib/FIFO ASCII read   header={'P1:'}  term=[13 10]  hold=Zero output if no new data  enable=off  maxsize=1024  outputtype=8 bit uint null terminated  sampletime=0.1
  LCM Output : Outport
  wires:
  LCM Input/1 -> FIFO ASCII read 1/1
  FIFO ASCII read 1/1 -> ASCII Decode 6/1
  Bus Creator4/1 -> LCM Output/1  "LCM Message"
  ASCII Decode 6/1 -> Bus Creator1/1  "X"
  ASCII Decode 6/2 -> Bus Creator1/2  "Y"
  ASCII Decode 6/3 -> Bus Creator1/3  "Psi"
  Bus Creator1/1 -> Bus Creator4/1  "Pose"
  ASCII Decode 6/4 -> Bus Creator2/1  "u"
  ASCII Decode 6/5 -> Bus Creator2/2  "v"
  Bus Creator2/1 -> Bus Creator4/2  "Velocity"
  ASCII Decode 6/7 -> Bus Creator3/1  "Roll"
  ASCII Decode 6/8 -> Bus Creator3/2  "Pitch"
  ASCII Decode 6/9 -> Bus Creator3/3  "Yaw"
  Bus Creator3/1 -> Bus Creator4/3  "Euler"
  Bus Creator5/1 -> Bus Creator4/4  "Port"
  Bus Creator6/1 -> Bus Creator4/5  "Stbd"
  ASCII Decode 6/12 -> Bus Creator6/1  "StThrust"
  ASCII Decode 6/13 -> Bus Creator6/2  "StAzimuth"
  ASCII Decode 6/10 -> Bus Creator5/1  "PtThrust"
  ASCII Decode 6/11 -> Bus Creator5/2  "PtAzimuth"
  ASCII Decode 6/14 -> Bus Creator4/6  "Start"
  ASCII Decode 6/15 -> Bus Creator4/7  "Elapsed"
  ASCII Decode 6/16 -> Data Type Conversion/1  "On/Off/RC/Auto"
  Data Type Conversion/1 -> Bus Creator4/8  "On/Off/RC/Auto"
  ASCII Decode 6/6 -> Bus Creator2/3  "r"

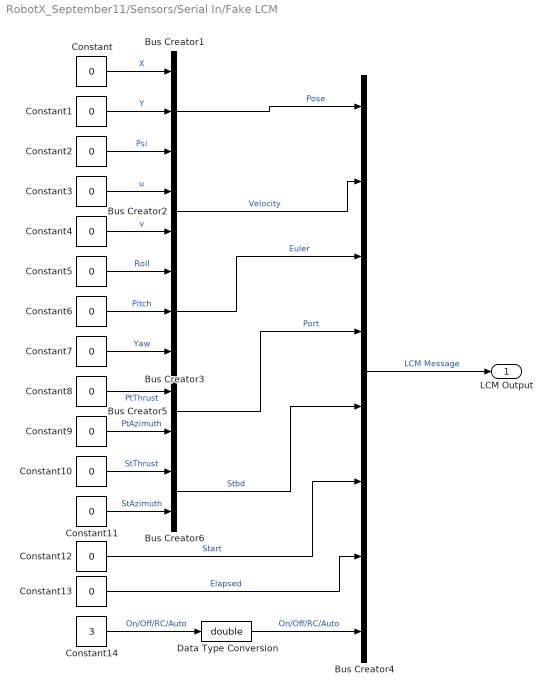
== system RobotX_September11/Sensors/Serial In/Fake LCM ==
  Bus Creator1 : BusCreator  Inputs=3
  Bus Creator2 : BusCreator  Inputs=2
  Bus Creator3 : BusCreator  Inputs=3
  Bus Creator4 : BusCreator  Inputs=8
  Bus Creator5 : BusCreator  Inputs=2
  Bus Creator6 : BusCreator  Inputs=2
  Constant{,1..13} (14 alike) : Constant  Value=0
  Constant14 : Constant  Value=3
  Data Type Conversion : DataTypeConversion  OutDataTypeStr=double
  LCM Output : Outport
  wires:
  Bus Creator4/1 -> LCM Output/1  "LCM Message"
  Constant/1 -> Bus Creator1/1  "X"
  Constant1/1 -> Bus Creator1/2  "Y"
  Constant2/1 -> Bus Creator1/3  "Psi"
  Bus Creator1/1 -> Bus Creator4/1  "Pose"
  Constant3/1 -> Bus Creator2/1  "u"
  Constant4/1 -> Bus Creator2/2  "v"
  Bus Creator2/1 -> Bus Creator4/2  "Velocity"
  Constant5/1 -> Bus Creator3/1  "Roll"
  Constant6/1 -> Bus Creator3/2  "Pitch"
  Constant7/1 -> Bus Creator3/3  "Yaw"
  Bus Creator3/1 -> Bus Creator4/3  "Euler"
  Bus Creator5/1 -> Bus Creator4/4  "Port"
  Bus Creator6/1 -> Bus Creator4/5  "Stbd"
  Constant10/1 -> Bus Creator6/1  "StThrust"
  Constant11/1 -> Bus Creator6/2  "StAzimuth"
  Constant8/1 -> Bus Creator5/1  "PtThrust"
  Constant9/1 -> Bus Creator5/2  "PtAzimuth"
  Constant12/1 -> Bus Creator4/6  "Start"
  Constant13/1 -> Bus Creator4/7  "Elapsed"
  Constant14/1 -> Data Type Conversion/1  "On/Off/RC/Auto"
  Data Type Conversion/1 -> Bus Creator4/8  "On/Off/RC/Auto"

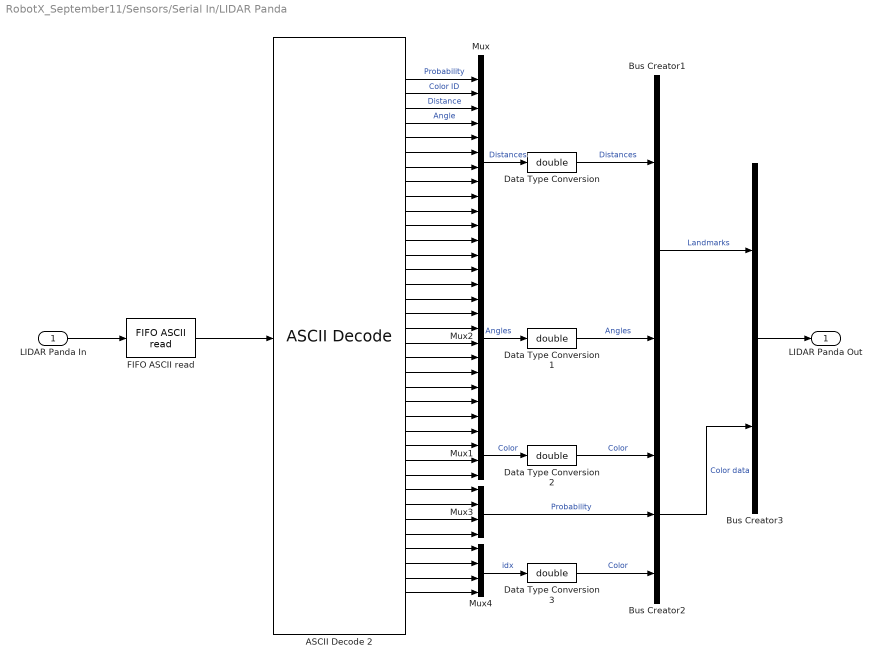
== system RobotX_September11/Sensors/Serial In/LIDAR Panda ==
  LIDAR Panda In : Inport
  ASCII Decode 2 : xpcseriallib/ASCII Decode   format=A:%d B:%d C:%d E:%d F:%d G:%d H:%d I:%d J:%d K:%d L:%d M:%d N:%d O:%d P:%d Q:%d R:%d S:%d T:%d U:%d V:%d W:%d X:%d C1:%d C2:%d C3:%d C4:%d P1:%f P2:%f P3:%f P4:%f I1:%d I2:%d I3:%d I4:%d \r\n  nvars=36  vartypes={}
  Bus Creator1 : BusCreator  Inputs=2
  Bus Creator2 : BusCreator  Inputs=3
  Bus Creator3 : BusCreator  Inputs=2
  Data Type Conversion{,1..3} (4 alike) : DataTypeConversion  OutDataTypeStr=double
  "FIFO ASCII read " : xpcseriallib/FIFO ASCII read   header={'A:'}  term=[13 10]  hold=Zero output if no new data  enable=off  maxsize=1024  outputtype=8 bit uint null terminated  sampletime=0.1
  Mux : Mux  Inputs=12
  Mux1 : Mux
  Mux2 : Mux  Inputs=12
  Mux3 : Mux
  Mux4 : Mux
  LIDAR Panda Out : Outport
  wires:
  LIDAR Panda In/1 -> "FIFO ASCII read "/1
  "FIFO ASCII read "/1 -> ASCII Decode 2/1
  ASCII Decode 2/3 -> Mux/3  "Distance"
  ASCII Decode 2/2 -> Mux/2  "Color ID"
  ASCII Decode 2/4 -> Mux/4  "Angle"
  ASCII Decode 2/1 -> Mux/1  "Probability"
  ASCII Decode 2/7 -> Mux/7
  ASCII Decode 2/10 -> Mux/10
  ASCII Decode 2/11 -> Mux/11
  ASCII Decode 2/6 -> Mux/6
  ASCII Decode 2/8 -> Mux/8
  ASCII Decode 2/9 -> Mux/9
  ASCII Decode 2/12 -> Mux/12
  ASCII Decode 2/5 -> Mux/5
  ASCII Decode 2/13 -> Mux2/1
  ASCII Decode 2/15 -> Mux2/3
  ASCII Decode 2/22 -> Mux2/10
  ASCII Decode 2/23 -> Mux2/11
  ASCII Decode 2/17 -> Mux2/5
  ASCII Decode 2/18 -> Mux2/6
  ASCII Decode 2/14 -> Mux2/2
  ASCII Decode 2/24 -> Mux2/12
  ASCII Decode 2/20 -> Mux2/8
  ASCII Decode 2/19 -> Mux2/7
  ASCII Decode 2/21 -> Mux2/9
  ASCII Decode 2/16 -> Mux2/4
  ASCII Decode 2/25 -> Mux1/1
  ASCII Decode 2/28 -> Mux1/4
  ASCII Decode 2/26 -> Mux1/2
  ASCII Decode 2/27 -> Mux1/3
  ASCII Decode 2/30 -> Mux3/2
  ASCII Decode 2/31 -> Mux3/3
  ASCII Decode 2/32 -> Mux3/4
  ASCII Decode 2/29 -> Mux3/1
  ASCII Decode 2/36 -> Mux4/4
  ASCII Decode 2/34 -> Mux4/2
  ASCII Decode 2/35 -> Mux4/3
  ASCII Decode 2/33 -> Mux4/1
  Mux/1 -> Data Type Conversion/1  "Distances"
  Mux2/1 -> Data Type Conversion1/1  "Angles"
  Mux1/1 -> Data Type Conversion2/1  "Color"
  Mux3/1 -> Bus Creator2/2  "Probability"
  Mux4/1 -> Data Type Conversion3/1  "idx"
  Bus Creator1/1 -> Bus Creator3/1  "Landmarks"
  Bus Creator2/1 -> Bus Creator3/2  "Color data"
  Bus Creator3/1 -> LIDAR Panda Out/1
  Data Type Conversion/1 -> Bus Creator1/1  "Distances"
  Data Type Conversion1/1 -> Bus Creator1/2  "Angles"
  Data Type Conversion2/1 -> Bus Creator2/1  "Color"
  Data Type Conversion3/1 -> Bus Creator2/3  "Color"

== matlab function RobotX_September11/Main FSM/Main Enabler ==
  data: taskSelector output; initEn output; gateEn output; parkEn output; reverseEn output; acSpinEn output; dodgeEn output; RCEn output; mainTask input; OnOffRCAuto input; initFin input; gateFin input; parkFin input; reverseFin input; acSpinFin input; dodgeFin input; termEn output
function [taskSelector,initEn,gateEn,parkEn,reverseEn,acSpinEn,dodgeEn,RCEn,...
    termEn] = taskEnabler(mainTask,OnOffRCAuto,initFin,gateFin,...
    parkFin,reverseFin,acSpinFin,dodgeFin)
%Written by Anderson Lebbad on July 19, 2013
%Last Edited: Edward Zhu on June 2, 2014
%   Substring search for task was written in
%   Case switches were redundant, combined with first set of if statements

%Changes the value of MainMode and the enablers for the tasks within the
%Main FSM.

% Initialize enable signals
RCEn = 0;
initEn = 0;
gateEn = 0;
parkEn = 0;
reverseEn = 0;
acSpinEn = 0;
dodgeEn = 0;
termEn = 0;

% Convert main task indicator to a string
mainTaskStr = char(mainTask);

% Adjust finished states based on user task selection (never skips
% initialization)
if ~isempty(strfind(mainTaskStr,'Park'))
    gateFin = 1;
elseif ~isempty(strfind(mainTaskStr,'Reverse'))
    gateFin = 1;
    parkFin = 1;
elseif ~isempty(strfind(mainTaskStr,'Spin'))
    gateFin = 1;
    parkFin = 1;
    reverseFin = 1;
elseif ~isempty(strfind(mainTaskStr,'Dodge'))
    gateFin = 1;
    parkFin = 1;
    reverseFin = 1;
    acSpinFin = 1;
end

% Set enable signals based on state completion
if initFin == 0
    initEn = 1;
    taskSelector = 1;
elseif OnOffRCAuto ~= 3
    RCEn = 1;
    taskSelector = 7;
elseif gateFin == 0
    gateEn = 1;
    taskSelector = 2;
elseif parkFin == 0
    parkEn = 1;
    taskSelector = 3;
elseif reverseFin == 0
    reverseEn = 1;
    taskSelector = 4;
elseif acSpinFin == 0
    dodgeEn = 1;
    taskSelector = 5;
elseif dodgeFin == 0
    dodgeEn = 1;
    taskSelector = 6;
else
    termEn = 1;
    taskSelector = 8;
end

== matlab function RobotX_September11/Main FSM/Gate/Calculate Times ==
  data: pts input; u input; Data output
function Data = calcTimes(pts, u)
%Written by Anderson Lebbad on August 9, 2014
%Last Edited:

%Calculates times for the boat to get to points for a trajectory, and
%formats Data for communication

%Initialize
Data = zeros(12,1);
traj = zeros(4,3);
traj(:,1:2) = pts;



for k = 2:4
    %Calculate distance to travel from last point
    distTravel = sqrt(sum((pts(k-1,:)-pts(k,:)).^2));
    %Assume 1m per second speed
    traj(k,3) = traj(k-1,3) + distTravel;
    %Add time based off initial velocity to get to first point past initial
    if k == 2
        traj(k,3) = traj(k,3) + 2.5*abs(2-u);
    end
end


%Output Data
for i=1:4
    for j = 1:3
        Data(3*(i-1)+j) = traj(i,j);
    end
end

== matlab function RobotX_September11/Sensors/Serial In/Data Update ==
  data: Valid input; ControlMode input; V output; C output; Data input; D1 output; D2 output; D3 output; D4 output; D5 output; D6 output; D7 output; D8 output; D9 output; D10 output; D11 output; D12 output; D13 output; D14 output; D15 output; D16 output; D17 output; D18 output; D19 output; D20 output; D21 output; D22 output; D23 output; D24 output
function [V,C,D1,D2,D3,D4,D5,D6,D7,D8,D9,D10,D11,D12,D13,D14,D15,D16,D17,...
    D18,D19,D20,D21,D22,D23,D24] = dataSplit(Valid,ControlMode,Data)
%Written by Anderson Lebbad on August 10, 2014
%Last Edited by: Anderson Lebbad on September 11, 2014

%This function splits the data vector into the twelve channels it is
%composed of for communication

persistent HoldData

if isempty(HoldData)
    HoldData = zeros(14,1);
end

if Valid == 1
    HoldData(1) = Valid;
    HoldData(2) = ControlMode;
    HoldData(3) = Data(1);
    HoldData(4) = Data(2);
    HoldData(5) = Data(3);
    HoldData(6) = Data(4);
    HoldData(7) = Data(5);
    HoldData(8) = Data(6);
    HoldData(9) = Data(7);
    HoldData(10) = Data(8);
    HoldData(11) = Data(9);
    HoldData(12) = Data(10);
    HoldData(13) = Data(11);
    HoldData(14) = Data(12);
    %     HoldData(15) = Data(13);
    %     HoldData(16) = Data(14);
    %     HoldData(17) = Data(15);
    %     HoldData(18) = Data(16);
    %     HoldData(19) = Data(17);
    %     HoldData(20) = Data(18);
    %     HoldData(21) = Data(19);
    %     HoldData(22) = Data(20);
    %     HoldData(23) = Data(21);
    %     HoldData(24) = Data(22);
    %     HoldData(25) = Data(23);
    %     HoldData(26) = Data(24);
    %     HoldData(15:26) = zeros(12,1);
end

V = HoldData(1);
C = HoldData(2);

if C == 0
    D1 = HoldData(3);
    D2 = HoldData(4);
    D3 = HoldData(5);
    D4 = (HoldData(6) - HoldData(3))/3 + HoldData(3);
    D5 = (HoldData(7) - HoldData(4))/3 + HoldData(4);
    D6 = (HoldData(8) - HoldData(5))/3 + HoldData(5);
    D7 = 2*(HoldData(6) - HoldData(3))/3 + HoldData(3);
    D8 = 2*(HoldData(7) - HoldData(4))/3 + HoldData(4);
    D9 = 2*(HoldData(8) - HoldData(5))/3 + HoldData(5);
    D10 = HoldData(6);
    D11 = HoldData(7);
    D12 = HoldData(8);
    D13 = (HoldData(9) - HoldData(6))/2 + HoldData(6);
    D14 = (HoldData(10) - HoldData(7))/2 + HoldData(7);
    D15 = (HoldData(11) - HoldData(8))/2 + HoldData(8);
    D16 = HoldData(9);
    D17 = HoldData(10);
    D18 = HoldData(11);
    D19 = (HoldData(12) - HoldData(9))/2 + HoldData(9);
    D20 = (HoldData(13) - HoldData(10))/2 + HoldData(10);
    D21 = (HoldData(14) - HoldData(11))/2 + HoldData(11);
    D22 = HoldData(12);
    D23 = HoldData(13);
    D24 = HoldData(14);
else
    D1 = HoldData(3);
    D2 = HoldData(4);
    D3 = HoldData(5);
    D4 = 0;
    D5 = 0;
    D6 = 0;
    D7 = 0;
    D8 = 0;
    D9 = 0;
    D10 = 0;
    D11 = 0;
    D12 = 0;
    D13 = 0;
    D14 = 0;
    D15 = 0;
    D16 = 0;
    D17 = 0;
    D18 = 0;
    D19 = 0;
    D20 = 0;
    D21 = 0;
    D22 = 0;
    D23 = 0;
    D24 = 0;
end

== matlab function RobotX_September11/Main FSM/Dodge/Dodge ==
  data: Finished output; time input; Valid output; X input; Y input; Psi input; Dist input; Angles input; pts output
function [Finished, Valid, pts] = Dodge(time,X,Y,Psi,Dist,Angles)
%Written by Anderson Lebbad on August 9, 2014
%Last Edited by:

%This function sends a forward trajectory (from the initial heading read
%into it) until a landmark is found. Once the landmark is found, a
%trajectory is written to dodge around it.

persistent HeldHeading hasFound finPt sample
if isempty(HeldHeading)
    HeldHeading = Psi;
    hasFound = 0;
    finPt = [0 0];
    sample = 50;
end

ts = 5;
dodgeLength = 15;
dodgeWidth = 5;
Finished = 0;
Valid = 0;
pts = zeros(4,2);
%Distance to object in meters
DistM = Dist/100;

%Set Valid bit. If it has been found in a previous timestep, the point is
%invalid, otherwise it is valid every increment of ts or if an object is
%found

%If no Landmark is found, navigate forward
if hasFound == 0
    %Initial pt
    pts(1,1) = X + 5*cos(HeldHeading*pi/180);
    pts(1,2) = Y + 5*sin(HeldHeading*pi/180);
    %Nothing found
    if Dist(1) == 0
        pts(2,1) = X + 10*cos(HeldHeading*pi/180);
        pts(2,2) = Y + 10*sin(HeldHeading*pi/180);
        pts(3,1) = X + 15*cos(HeldHeading*pi/180);
        pts(3,2) = Y + 15*sin(HeldHeading*pi/180);
        pts(4,1) = X + 20*cos(HeldHeading*pi/180);
        pts(4,2) = Y + 20*sin(HeldHeading*pi/180);
        %Only flip valid bit every ts (seconds)
        sample = sample + 1;
        if sample >= 50
            Valid = 1;
            sample = 0;
        end
    %Something found
    else
        %Absolute Heading of object relative to boat's position
        landmarkHeading = mod((Psi + Angles(1)),360);
        lmHeadingRad = landmarkHeading*pi/180;
        %Navigate to it
        pts(2,1) = X + DistM(1)*cos(lmHeadingRad) - dodgeWidth*sin(lmHeadingRad);
        pts(2,2) = Y + DistM(1)*sin(lmHeadingRad) + dodgeWidth*cos(lmHeadingRad);
        pts(3,1) = X + (DistM(1) + dodgeLength)*cos(lmHeadingRad);
        pts(3,2) = Y + (DistM(1) + dodgeLength)*sin(lmHeadingRad);
        pts(4,1) = X + (DistM(1) + 2*dodgeLength)*cos(lmHeadingRad);
        pts(4,2) = Y + (DistM(1) + 2*dodgeLength)*sin(lmHeadingRad);
        finPt = pts(3,:);
        %Flip valid if found
        Valid = 1;
        %Tag object as having been found
        hasFound = 1;
    end
end

%Check to see how far the current pose is from the final point in the
%trajectory
range = sqrt(sum((finPt - [X Y]).^2));
if range <= 3 && hasFound == 1
    Finished = 1;
end

%Output ptsHeld as pts
pts = pts;

end

== matlab function RobotX_September11/Main FSM/Acoustic Spin/Spin ==
  data: X input; Data output; Y input; Psi input
function Data = Spin(X,Y,Psi)
%Written by Anderson Lebbad on August 9, 2014
%Last Edited:

%This function passes the current pose data with a heading offset as the
%desired pose for the station keeping controller to use.

persistent holdPose

if isempty(holdPose)
    holdPose = [X Y Psi];
end

%Initialize Data variable
Data = zeros(12,1);

%Angular offset (indirect rate control)
offset = 30;

holdPose(3) = Psi + offset;

%Set desired pose
Data(1) = holdPose(1);
Data(2) = holdPose(2);
Data(3) = holdPose(3);
